simulink model "tire_estimator"  (R2024b)
settings: Solver=FixedStepAuto  StartTime=0.0  StopTime=10.0  RelTol=1e-3
settings Model: Creator=lukec  LastModifiedBy=lukec
settings OptimizationCC: DefaultParameterBehavior=Inlined  EnhancedBackFolding=on  PassReuseOutputArgsAs=Individual arguments  ZeroExternalMemoryAtStartup=off  ZeroInternalMemoryAtStartup=off  OptimizeBlockOrder=speed  DifferentSizesBufferReuse=on  OptimizationCustomize=off  EfficientTunableParamExpr=on
settings DebuggingCC: ParameterTunabilityLossMsg=error
settings HardwareCC: ProdBitPerPointer=32  ProdBitPerSizeT=32  ProdBitPerPtrDiffT=32  ProdLargestAtomicInteger=Long  ProdLargestAtomicFloat=Double  ProdWordSize=32  ProdHWDeviceType=ARM Compatible->ARM Cortex-M
settings SFSimCC: MATLABDynamicMemAlloc=off
settings RTWCC: Description=Embedded Coder  SystemTargetFile=ert.tlc  GenCodeOnly=on  PackageGeneratedCodeAndArtifacts=on  TemplateMakefile=ert_default_tmf  Toolchain=CMake  TargetLang=C++  HalideCodeGeneration=on
settings CodeAppCC: ForceParamTrailComments=on  IgnoreCustomStorageClasses=off  MaxIdLength=255  OperatorAnnotations=on  SimulinkDataObjDesc=on  SFDataObjDesc=on  InsertBlockDesc=on
settings ERTTargetCC: TargetLangStandard=C++17 (ISO)  CodeInterfacePackaging=C++ class  RootIOFormat=Structure reference  ERTCustomFileTemplate=example_file_process.tlc  ArrayContainerType=std::array

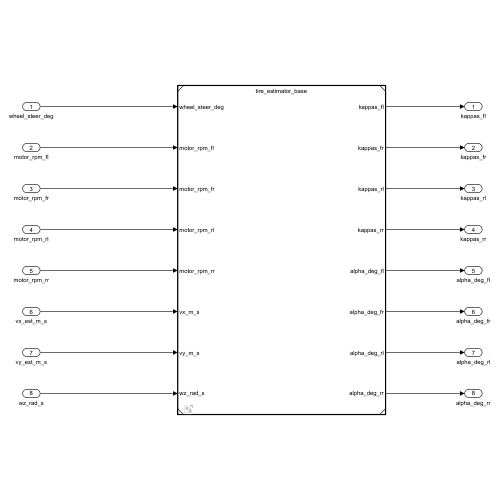
[thumbnail: Simulink's stored preview of the top-level diagram]
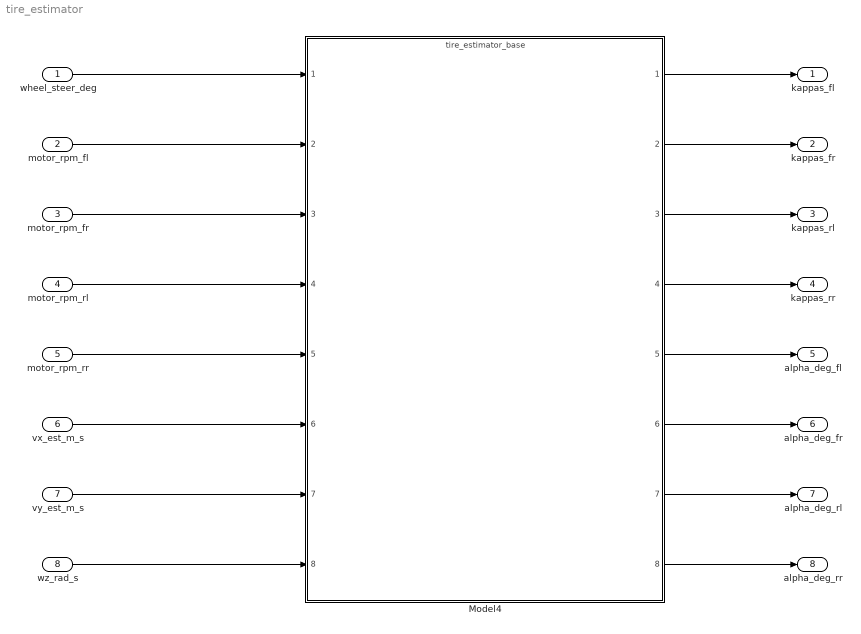
== system tire_estimator ==
  wheel_steer_deg : Inport
  motor_rpm_fl : Inport  Port=2
  motor_rpm_fr : Inport  Port=3
  motor_rpm_rl : Inport  Port=4
  motor_rpm_rr : Inport  Port=5
  vx_est_m_s : Inport  Port=6
  vy_est_m_s : Inport  Port=7
  wz_rad_s : Inport  Port=8
  Model4 : ModelReference  ModelNameDialog=tire_estimator_base.slx  SimulationMode=Normal  ModelReferenceVersion=1.6
  kappas_fl : Outport
  kappas_fr : Outport  Port=2
  kappas_rl : Outport  Port=3
  kappas_rr : Outport  Port=4
  alpha_deg_fl : Outport  Port=5
  alpha_deg_fr : Outport  Port=6
  alpha_deg_rl : Outport  Port=7
  alpha_deg_rr : Outport  Port=8
  wires:
  wheel_steer_deg/1 -> Model4/1
  motor_rpm_fl/1 -> Model4/2
  motor_rpm_fr/1 -> Model4/3
  motor_rpm_rl/1 -> Model4/4
  vx_est_m_s/1 -> Model4/6
  motor_rpm_rr/1 -> Model4/5
  vy_est_m_s/1 -> Model4/7
  wz_rad_s/1 -> Model4/8
  Model4/1 -> kappas_fl/1
  Model4/2 -> kappas_fr/1
  Model4/3 -> kappas_rl/1
  Model4/4 -> kappas_rr/1
  Model4/5 -> alpha_deg_fl/1
  Model4/6 -> alpha_deg_fr/1
  Model4/7 -> alpha_deg_rl/1
  Model4/8 -> alpha_deg_rr/1
